simulink model "BuckBoost1"  (Simulink 8.0)
settings: Solver=FixedStepDiscrete  StartTime=0.0  StopTime=5  FixedStep=1e-5  RelTol=1e-3
undefined symbols (not defined in the file): Imax, R, Ts, Vin
libraries: powerlib x12, powerlib_extras x2
settings Model: Creator=zxn  LastModifiedBy=Harri
settings DataIOCC: SignalLoggingSaveFormat=ModelDataLogs
settings DebuggingCC: FcnCallInpInsideContextMsg=UseLocalSettings
settings GRTTargetCC: CombineOutputUpdateFcns=off  GRTInterface=on

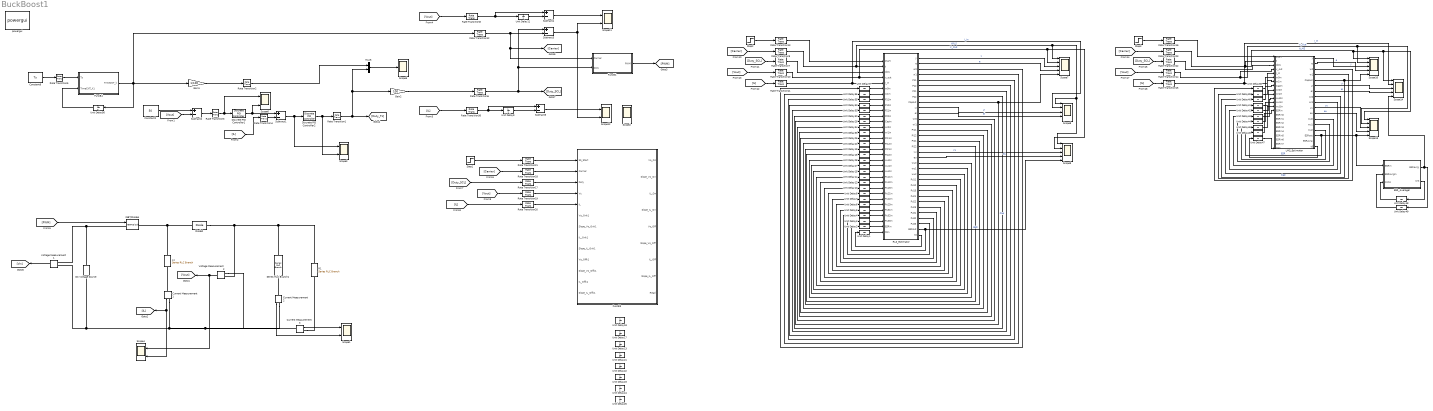
== system BuckBoost1 ==
  Constant2 : Constant  Value=50
  Constant6 : Constant  Value=Ts
  Current Measurement1 : powerlib/Measurements/Current Measurement  PhasorSimulation=off  OutputType=Complex  PSBequivalent=0
  Current Measurement2 : powerlib/Measurements/Current Measurement  PhasorSimulation=off  OutputType=Complex  PSBequivalent=0
  Current Measurement3 : powerlib/Measurements/Current Measurement  PhasorSimulation=off  OutputType=Complex  PSBequivalent=0
  DC Voltage Source : powerlib/Electrical Sources/DC Voltage Source  Amplitude=Vin  Measurements=None
  Diode2 : powerlib/Power Electronics/Diode  Ron=0.001  Lon=0  Vf=0.8  IC=0  UseSnubber=off  Rs=inf  Cs=inf  Measurements=off
  Discrete PID Controller1 : powerlib_extras/Discrete  Control Blocks/Discrete PID Controller  Kp=1.4  Ki=0.4  Kd=0  TcD=0  Par_Limits=[1 -1]*Imax  Init=0  Ts=Ts
  Discrete PID Controller2 : powerlib_extras/Discrete  Control Blocks/Discrete PID Controller  Kp=30e-3  Ki=50e-3  Kd=0  TcD=0  Par_Limits=[1 -1]*0.9  Init=0  Ts=Ts
  ESR_Averager : MATLAB Function  TreatAsAtomicUnit=on
  FuncB1 : MATLAB Function  TreatAsAtomicUnit=on
  FuncB3 : MATLAB Function  TreatAsAtomicUnit=on
  FuncB4 : MATLAB Function  TreatAsAtomicUnit=on
  Gain1 : Gain  Gain=1/100
  Gain2 : Gain  Gain=100
  IGBT/Diode4 : powerlib/Power Electronics/IGBT//Diode  Ron=1e-3  Rs=1e5  Cs=inf  Measurements=off
  L1 : powerlib/Elements/Series RLC Branch  LConnTagsString=__new0  RConnTagsString=__new0  BranchType=L  Resistance=1  Inductance=5e-3  SetiL0=off  InitialCurrent=0  Capacitance=1e-6  Setx0=off  InitialVoltage=0  Measurements=None
  LMS_Estimator : MATLAB Function  TreatAsAtomicUnit=on
  Mux5 : Mux  Inputs=2
  R1 : powerlib/Elements/Series RLC Branch  LConnTagsString=__new0  RConnTagsString=__new0  BranchType=R  Resistance=R  Inductance=1e-3  SetiL0=off  InitialCurrent=0  Capacitance=1e-6  Setx0=off  InitialVoltage=0  Measurements=None
  RLS_Estimator : MATLAB Function  TreatAsAtomicUnit=on
  Rate Transition{1..2,6..23,30} (21 alike) : RateTransition  OutPortSampleTime=1e-5
  Rate Transition3 : RateTransition  OutPortSampleTime=Ts
  Rate Transition4 : RateTransition  OutPortSampleTime=Ts
  Rate Transition5 : RateTransition  X0=Ts  OutPortSampleTime=1e-5
  Scope{1,3..4,6,11..12} (6 alike) : Scope  NumInputPorts=2
      Scope1 settings: TickLabels=on  TimeRange=10  YMin=210~0  YMax=320~47.5  SaveName=var1
      Scope11 settings: TickLabels=on  TimeRange=5  YMin=-0.06~-40  YMax=0.07~65  SaveName=var10  MaxDataPoints=1000000
      Scope12 settings: TickLabels=on  TimeRange=5  YMin=-0.011~-40  YMax=0.01~65  SaveName=var13  MaxDataPoints=1000000
      Scope3 settings: TickLabels=on  TimeRange=1.5  YMin=0.5~0  YMax=0.605~1  SaveName=var4
      Scope4 settings: TickLabels=on  YMin=41.5~2.4  YMax=50~4.3  SaveName=var
      Scope6 settings: TickLabels=on  TimeRange=1.5  YMin=0.5~0  YMax=0.605~1  SaveName=var2
  Scope{7..10,13..14} (6 alike) : Scope  NumInputPorts=5
      Scope10 settings: TickLabels=on  TimeRange=5  YMin=-0.011~-40~-5~-5~-5  YMax=0.01~65~5~5~5  SaveName=var9  MaxDataPoints=1000000
      Scope13 settings: TickLabels=on  TimeRange=5  YMin=-0.011~-40~-5~-5~-5  YMax=0.01~65~5~5~5  SaveName=var11  MaxDataPoints=1000000
      Scope14 settings: TickLabels=on  TimeRange=5  YMin=-0.011~-40~-5~-5~0  YMax=0.01~65~5~5~125  SaveName=var12  MaxDataPoints=1000000
      Scope7 settings: TickLabels=on  TimeRange=5  YMin=-0.011~-40~-5~-5~-5  YMax=0.01~65~5~5~5  SaveName=var6  MaxDataPoints=1000000
      Scope8 settings: TickLabels=on  TimeRange=5  YMin=-0.011~-40~-5~-5~-5  YMax=0.01~65~5~5~5  SaveName=var7  MaxDataPoints=1000000
      Scope9 settings: TickLabels=on  TimeRange=5  YMin=-0.011~-40~-5~-5~-5  YMax=0.01~65~5~5~5  SaveName=var8  MaxDataPoints=1000000
  Scope2 : Scope  NumInputPorts=4
      settings: TickLabels=on  TimeRange=5  YMin=-0.011~-40~-5~-5  YMax=0.01~65~5~5  SaveName=var3  MaxDataPoints=1000000
  Scope5 : Scope
      settings: TickLabels=on  TimeRange=1.5  YMin=0.5  YMax=0.605  SaveName=var5  MaxDataPoints=100000
  Series RLC Branch1 : powerlib/Elements/Series RLC Branch  LConnTagsString=__new0  RConnTagsString=__new0  BranchType=RC  Resistance=80e-3*1  Inductance=1e-3  SetiL0=off  InitialCurrent=0  Capacitance=1e-3*1.75  Setx0=off  InitialVoltage=500  Measurements=None
  Step1 : Step  Time=3.3  SampleTime=0
  Step2 : Step  Time=3.3  SampleTime=0
  Step3 : Step  Time=3.3  SampleTime=0
  Subtract1 : Sum  Inputs=+-  SampleTime=Ts
  Subtract{2..5} (4 alike) : Sum  Inputs=+-
  Unit Delay{1..2,4..6,8..13,15,17..25,27..29,31..34,36..49,56} (43 alike) : UnitDelay  SampleTime=1e-5
  Unit Delay{3,7,14,16,26,30,35} (7 alike) : UnitDelay  InitialCondition=100  SampleTime=1e-5
  Voltage Measurement1 : powerlib/Measurements/Voltage Measurement  PhasorSimulation=off  OutputType=Complex  PSBequivalent=0
  Voltage Measurement2 : powerlib/Measurements/Voltage Measurement  PhasorSimulation=off  OutputType=Complex  PSBequivalent=0
  powergui : powerlib/powergui  Priority=2  SimulationMode=Discrete  SolverType=Tustin  SampleTime=1e-5  frequency=60  SPID=off  DisableSnubberDevices=off  DisableRonSwitches=off  DisableVfSwitches=off  SwTol=0  Interpol=off  DisplayEquations=off  FunctionMessages=off  frequencyindice=0  Pbase=100e6  ErrMax=1e-4  Iterations=50  UnitsV=kV  UnitsW=MW  echomessages=off  HookPort=off  EnableUseOfTLC=off  x0status=blocks  RestoreLinks=warning  ResistiveCurrentMeasurement=off  Frange=[0:2:500]  Ylog=off  Xlog=off  ShowGrid=off  save=off  variable=ZData  structure=ScopeData  ZoomFFT=on  StartTime=0.0  cycles=1  DisplayStyle=1  fundamental=60  FreqAxis=off  MaxFrequency=8000  frequencyindicesteady=1  RmsSteady=1  display=off  Ts=0  methode=off
  wires:
  Constant2/1 -> Subtract2/1
  Subtract2/1 -> Rate Transition3/1
  Voltage Measurement2/1 -> Scope4/1, [Vout]
  Current Measurement1/1 -> [IL], Scope4/2
  Current Measurement3/1 -> Scope1/1
  Current Measurement2/1 -> Scope1/2
  Rate Transition2/1 -> Mux5/1
  Rate Transition3/1 -> Discrete PID Controller1/1, Scope6/1
  Discrete PID Controller1/1 -> Subtract1/1, Scope6/2
  Subtract1/1 -> Discrete PID Controller2/1, Scope3/1
  Rate Transition4/1 -> Subtract1/2
  [IL] -> Rate Transition4/1
  [Vout] -> Subtract2/2
  Discrete PID Controller2/1 -> Rate Transition1/1, Scope3/2
  Rate Transition1/1 -> Mux5/2, Gain2/1, [Duty_Ts]
  Mux5/1 -> Scope5/1
  Rate Transition6/1 -> [Duty_SCL], Subtract3/1, FuncB1/2(Duty)
  Rate Transition8/1 -> Unit Delay11/1, Subtract4/1
  [PWM] -> IGBT/Diode4/1
  Voltage Measurement1/1 -> [Vin]
  Rate Transition5/1 -> FuncB4/1(Ts)
  Constant6/1 -> Rate Transition5/1
  Unit Delay56/1 -> FuncB4/2(TimeCNT_k1)
  FuncB4/1(TimeCNT_k) -> Unit Delay56/1, Gain1/1, Rate Transition12/1
  Gain1/1 -> Rate Transition2/1
  Gain2/1 -> Rate Transition6/1
  Subtract3/1 -> Scope11/2, Scope12/2
  Rate Transition12/1 -> Subtract3/2, [Carrier], FuncB1/1(Carrier)
  Unit Delay11/1 -> Subtract4/2
  Subtract4/1 -> Scope11/1
  [Vout] -> Rate Transition8/1
  [Carrier] -> Rate Transition18/1
  [Duty_SCL] -> Rate Transition17/1
  Step1/1 -> Rate Transition21/1
  [IL] -> Rate Transition20/1
  [Vout] -> Rate Transition19/1
  FuncB1/1(PWM) -> [PWM]
  Rate Transition21/1 -> FuncB3/1(SS_Start)
  Rate Transition18/1 -> FuncB3/2(Carrier)
  Rate Transition17/1 -> FuncB3/3(Duty)
  Rate Transition19/1 -> FuncB3/4(Vc)
  Rate Transition20/1 -> FuncB3/5(IL)
  [IL] -> Rate Transition30/1
  Unit Delay9/1 -> Subtract5/2
  Rate Transition30/1 -> Unit Delay9/1, Subtract5/1
  Subtract5/1 -> Scope12/1
  [Carrier] -> Rate Transition9/1
  [Duty_SCL] -> Rate Transition7/1
  Step2/1 -> Rate Transition13/1
  [IL] -> Rate Transition11/1
  [Vout] -> Rate Transition10/1
  Rate Transition9/1 -> Scope7/1, Scope8/1, Scope9/1, RLS_Estimator/2(t)  "tRLS"
  Rate Transition7/1 -> RLS_Estimator/3(duty)
  Rate Transition10/1 -> Scope7/2, Scope9/2, RLS_Estimator/4(v_out)  "V_Out"
  Rate Transition11/1 -> Scope8/2, RLS_Estimator/5(i_in)  "I_In"
  Rate Transition13/1 -> RLS_Estimator/1(start)
  Unit Delay1/1 -> RLS_Estimator/32(t0in)
  Unit Delay2/1 -> RLS_Estimator/31(ESRin)
  Unit Delay3/1 -> RLS_Estimator/30(Pu33in)
  Unit Delay4/1 -> RLS_Estimator/29(Pu32in)
  Unit Delay5/1 -> RLS_Estimator/28(Pu31in)
  Unit Delay6/1 -> RLS_Estimator/27(Pu23in)
  Unit Delay7/1 -> RLS_Estimator/26(Pu22in)
  Unit Delay8/1 -> RLS_Estimator/25(Pu21in)
  Unit Delay10/1 -> RLS_Estimator/24(Pu13in)
  Unit Delay12/1 -> RLS_Estimator/23(Pu12in)
  Unit Delay14/1 -> RLS_Estimator/22(Pu11in)
  Unit Delay15/1 -> RLS_Estimator/21(wu2in)
  Unit Delay27/1 -> RLS_Estimator/20(wu1in)
  Unit Delay28/1 -> RLS_Estimator/19(wu0in)
  Unit Delay16/1 -> RLS_Estimator/18(Pi22in)
  Unit Delay19/1 -> RLS_Estimator/17(Pi21in)
  Unit Delay20/1 -> RLS_Estimator/16(Pi12in)
  Unit Delay26/1 -> RLS_Estimator/15(Pi11in)
  Unit Delay33/1 -> RLS_Estimator/14(wi1in)
  Unit Delay34/1 -> RLS_Estimator/13(wi0in)
  Unit Delay29/1 -> RLS_Estimator/12(Capin)
  Unit Delay30/1 -> RLS_Estimator/11(P22in)
  Unit Delay31/1 -> RLS_Estimator/10(P21in)
  Unit Delay32/1 -> RLS_Estimator/9(P12in)
  Unit Delay35/1 -> RLS_Estimator/8(P11in)
  Unit Delay36/1 -> RLS_Estimator/7(w1in)
  Unit Delay37/1 -> RLS_Estimator/6(w0in)
  RLS_Estimator/33(t0) -> Unit Delay1/1
  RLS_Estimator/32(ESRout) -> Unit Delay2/1, Scope9/5  "ESR"
  RLS_Estimator/31(Pu33) -> Unit Delay3/1
  RLS_Estimator/30(Pu32) -> Unit Delay4/1
  RLS_Estimator/29(Pu31) -> Unit Delay5/1
  RLS_Estimator/28(Pu23) -> Unit Delay6/1
  RLS_Estimator/27(Pu22) -> Unit Delay7/1
  RLS_Estimator/26(Pu21) -> Unit Delay8/1
  RLS_Estimator/25(Pu13) -> Unit Delay10/1
  RLS_Estimator/24(Pu12) -> Unit Delay12/1
  RLS_Estimator/23(Pu11) -> Unit Delay14/1
  RLS_Estimator/22(wu2) -> Unit Delay15/1
  RLS_Estimator/21(wu1) -> Unit Delay27/1
  RLS_Estimator/20(wu0) -> Unit Delay28/1
  RLS_Estimator/17(Pi22) -> Unit Delay16/1
  RLS_Estimator/16(Pi21) -> Unit Delay19/1
  RLS_Estimator/15(Pi12) -> Unit Delay20/1
  RLS_Estimator/14(Pi11) -> Unit Delay26/1
  RLS_Estimator/13(wi1) -> Unit Delay33/1
  RLS_Estimator/12(wi0) -> Unit Delay34/1
  RLS_Estimator/9(Capout) -> Unit Delay29/1, Scope7/5  "Cap"
  RLS_Estimator/8(P22) -> Unit Delay30/1
  RLS_Estimator/7(P21) -> Unit Delay31/1
  RLS_Estimator/6(P12) -> Unit Delay32/1
  RLS_Estimator/5(P11) -> Unit Delay35/1
  RLS_Estimator/4(w1) -> Unit Delay36/1
  RLS_Estimator/3(w0) -> Unit Delay37/1
  RLS_Estimator/2(e) -> Scope7/4  "e"
  RLS_Estimator/1(y) -> Scope7/3  "y"
  RLS_Estimator/10(yi) -> Scope8/3  "yi"
  RLS_Estimator/11(ei) -> Scope8/4  "ei"
  RLS_Estimator/18(yu) -> Scope9/3  "yu"
  RLS_Estimator/19(eu) -> Scope9/4  "eu"
  [Carrier] -> Rate Transition23/1
  [Duty_SCL] -> Rate Transition22/1
  Step3/1 -> Rate Transition16/1
  [IL] -> Rate Transition15/1
  [Vout] -> Rate Transition14/1
  Rate Transition23/1 -> Scope14/1, Scope13/1, Scope10/1, LMS_Estimator/2(t)  "tLMS"
  Rate Transition22/1 -> LMS_Estimator/3(duty)
  Rate Transition14/1 -> Scope10/2, Scope13/2, LMS_Estimator/4(v_out)  "V_Out"
  Rate Transition15/1 -> Scope14/2, LMS_Estimator/5(i_in)  "I_In"
  Rate Transition16/1 -> LMS_Estimator/1(start)
  Unit Delay47/1 -> LMS_Estimator/23(t0in)
  Unit Delay46/1 -> LMS_Estimator/14(ESRin)
  Unit Delay45/1 -> LMS_Estimator/13(wu2in)
  Unit Delay44/1 -> LMS_Estimator/12(wu1in)
  Unit Delay43/1 -> LMS_Estimator/11(wu0in)
  Unit Delay42/1 -> LMS_Estimator/10(wi1in)
  Unit Delay41/1 -> LMS_Estimator/9(wi0in)
  Unit Delay40/1 -> LMS_Estimator/8(Capin)
  Unit Delay39/1 -> LMS_Estimator/7(w1in)
  Unit Delay38/1 -> LMS_Estimator/6(w0in)
  LMS_Estimator/17(t0) -> Unit Delay47/1
  LMS_Estimator/15(ESRout) -> Unit Delay46/1, ESR_Averager/1(ESRin), Scope13/5  "ESR"
  LMS_Estimator/14(wu2) -> Unit Delay45/1
  LMS_Estimator/13(wu1) -> Unit Delay44/1
  LMS_Estimator/12(wu0) -> Unit Delay43/1
  LMS_Estimator/9(wi1) -> Unit Delay42/1
  LMS_Estimator/8(wi0) -> Unit Delay41/1
  LMS_Estimator/4(w1) -> Unit Delay39/1
  LMS_Estimator/3(w0) -> Unit Delay38/1
  LMS_Estimator/1(y) -> Scope10/3  "y"
  LMS_Estimator/2(e) -> Scope10/4  "e"
  LMS_Estimator/5(Capout) -> Unit Delay40/1, Scope10/5  "Cap"
  LMS_Estimator/6(yi) -> Scope14/3  "yi"
  LMS_Estimator/7(ei) -> Scope14/4  "ei"
  LMS_Estimator/11(eu) -> Scope13/4  "eu"
  LMS_Estimator/10(yu) -> Scope13/3  "yu"
  ESR_Averager/2(Cnt) -> Unit Delay48/1
  Unit Delay48/1 -> ESR_Averager/3(CntIn)
  ESR_Averager/1(ESRavrg) -> Scope14/5, Unit Delay49/1
  Unit Delay49/1 -> ESR_Averager/2(ESRavrgIn)
  connections:
  DC Voltage Source/RConn1 -- IGBT/Diode4/LConn1 -- Voltage Measurement1/LConn1
  Diode2/RConn1 -- IGBT/Diode4/RConn1 -- L1/RConn1
  Current Measurement3/LConn1 -- Current Measurement2/RConn1 -- Voltage Measurement2/LConn1 -- Current Measurement1/RConn1 -- DC Voltage Source/LConn1 -- Voltage Measurement1/LConn2
  Current Measurement1/LConn1 -- L1/LConn1
  Diode2/LConn1 -- R1/RConn1 -- Series RLC Branch1/RConn1 -- Voltage Measurement2/LConn2
  Current Measurement2/LConn1 -- Series RLC Branch1/LConn1
  Current Measurement3/RConn1 -- R1/LConn1

== matlab function RLS_Estimator ==
  data: start input double; t input double; duty input double; v_out input double; i_in input double; w0in input double; w1in input double; P11in input double; P12in input double; P21in input double; P22in input double; Capin input double; y output double; e output double; w0 output double; w1 output double; P11 output double; P12 output double; P21 output double; P22 output double; Capout output double; wi0in input double; wi1in input double; Pi11in input double; Pi12in input double; Pi21in input double; Pi22in input double; wu0in input double; wu1in input double; wu2in input double; Pu11in input double; Pu12in input double; Pu13in input double; Pu21in input double; Pu22in input double; Pu23in input double; Pu31in input double; Pu32in input double; Pu33in input double; ESRin input double; t0in input double; yi output double; ei output double; wi0 output double; wi1 output double; Pi11 output double; Pi12 output double; Pi21 output double; Pi22 output double; yu output double; eu output double; wu0 output double; wu1 output double; wu2 output double; Pu11 output double; Pu12 output double; Pu13 output double; Pu21 output double; Pu22 output double; Pu23 output double; Pu31 output double; Pu32 output double; Pu33 output double; ESRout output double; t0 output double
function [y, e, w0, w1, P11, P12, P21, P22, Capout, ...
    yi, ei, wi0, wi1, Pi11, Pi12, Pi21, Pi22, ...
    yu, eu, wu0, wu1, wu2, Pu11, Pu12, Pu13, Pu21, Pu22, Pu23, Pu31, Pu32, Pu33, ESRout, ...
    t0]  = ...
    Est_RLS(start,t,duty,v_out,i_in, ...
    w0in, w1in, P11in, P12in, P21in, P22in, Capin, ...
    wi0in, wi1in, Pi11in, Pi12in, Pi21in, Pi22in, ...
    wu0in, wu1in, wu2in, Pu11in, Pu12in, Pu13in, Pu21in, Pu22in, Pu23in, Pu31in, Pu32in, Pu33in, ESRin, ...
    t0in)
%#codegen

% *** Time Partition ******************************************************
sampling_time = 1e-5;% 1e-6;

offset = t - duty;

OFFSET_ON_START_abs = 0+5; % for t
OFFSET_ON_END_rel = -5; % for offset
OFFSET_OFF_START_rel = 5; % for offset
OFFSET_OFF_END_abs = 90+5; % for t
% --- end of Time Partition -----------------------------------------------

% *** Init ****************************************************************
lambda = 0.6;
% good for change: 0.7; not good with change: 0.999;
delta = 1/100;

% <<~~~ uON(t) = w0 + w1*t ~~~~~~~~~~~~~~~~~~~~~~~~~~~~~~~~~~~~~~~~~~~~~~>>

% ... estimator output ...
y = 0.0;
e = 0.0;

% ... inputs ...
u = transpose(zeros(1,2));
u(1) = 1;
u(2) = t;

% ... coefficients ...
w = zeros(2,1);
w(1) = w0in;
w(2) = w1in;
w0 = w0in; w1 = w1in;

% ... algorithm specific tools ...
P = eye(2) / delta;
P(1,1) = P11in; P(1,2) = P12in;
P(2,1) = P21in; P(2,2) = P22in;
%NOTE: in "delay unit" blocks, set:
% P11in and P22in --> 100 (as per 'delta')
% P12in and P21in --> 0 (since "eye" matrix)
P11 = P11in; P12 = P12in;
P21 = P21in; P22 = P22in;

% <<~~~ iLOFF(t) = wi0 + wi1*t ~~~~~~~~~~~~~~~~~~~~~~~~~~~~~~~~~~~~~~~~~~>>

% ... estimator output ...
yi = 0.0;
ei = 0.0;

% ... inputs ...
% REUSE

% ... coefficients ...
wi = zeros(2,1);
wi(1) = wi0in;
wi(2) = wi1in;
wi0 = wi0in; wi1 = wi1in;

% ... algorithm specific tools ...
Pi = eye(2) / delta;
Pi(1,1) = Pi11in; Pi(1,2) = Pi12in;
Pi(2,1) = Pi21in; Pi(2,2) = Pi22in;
%NOTE: in "delay unit" blocks, set:
% P11in and P22in --> 100 (as per 'delta')
% P12in and P21in --> 0 (since "eye" matrix)
Pi11 = Pi11in; Pi12 = Pi12in;
Pi21 = Pi21in; Pi22 = Pi22in;

% <<~~~ uON(t) = wu0 + wu1*t + wu2*t^2 ~~~~~~~~~~~~~~~~~~~~~~~~~~~~~~~~~~>>

% ... estimator output ...
yu = 0.0;
eu = 0.0;

% ... inputs ...
uu = transpose(zeros(1,3));
uu(1) = 1;
uu(2) = t;
uu(3) = t*t;

% ... coefficients ...
wu = zeros(3,1);
wu(1) = wu0in;
wu(2) = wu1in;
wu(3) = wu2in;
wu0 = wu0in; wu1 = wu1in; wu2 = wu2in;

% ... algorithm specific tools ...
Pu = eye(3) / delta;
% TODO: remove P(i,j) with i!=j...
Pu(1,1) = Pu11in; Pu(1,2) = Pu12in; Pu(1,3) = Pu13in;
Pu(2,1) = Pu21in; Pu(2,2) = Pu22in; Pu(2,3) = Pu23in;
Pu(3,1) = Pu31in; Pu(3,2) = Pu32in; Pu(3,3) = Pu33in;
%NOTE: in "delay unit" blocks, set:
% P11in and P22in --> 100 (as per 'delta')
% P12in and P21in --> 0 (since "eye" matrix)
Pu11 = Pu11in; Pu12 = Pu12in; Pu13 = Pu13in;
Pu21 = Pu21in; Pu22 = Pu22in; Pu23 = Pu23in;
Pu31 = Pu31in; Pu32 = Pu32in; Pu33 = Pu33in;

% --- end of Init ---------------------------------------------------------

% *** Misc. ***************************************************************

Capout = Capin;
ESRout = ESRin;
t0 = t0in;

% --- end of Misc. --------------------------------------------------------

noiseAmp = 0; % rand : [0,1]

if(start==1)
    % *** State: ON *******************************************************
    if(t > OFFSET_ON_START_abs && offset < OFFSET_ON_END_rel) % ON
        % estimate the "C"
        if(t > OFFSET_ON_START_abs && t<= OFFSET_ON_START_abs+2)
            t0 = t;
        else
            % --- start of RLS for uON(t) ---
            %u(2) = t - t0; NOTE: RLS do not require this kind of offsetting!
            u(2) = (t - t0) * sampling_time; %NOTE: not necessary to offset!
            k = ( (P*u) / (1 + (u' * P * u) / lambda) ) / lambda;
            y = w' * u;
            %e = v_out - y;
            e = (v_out + (noiseAmp*rand)) - y;

            w = w + k*e;
            w0 = w(1); w1 = w(2);

            P = ( P - k * u' * P ) / lambda;
            P11 = P(1,1); P12 = P(1,2);
            P21 = P(2,1); P22 = P(2,2);
            % --- end of RLS for uON(t) ---
        end
    end
    if(offset >= OFFSET_ON_END_rel && offset <= OFFSET_ON_END_rel+1)
        Capout = -w0/w1/30;%*sampling_time;%R=30
    end
    % --- end State: ON ---------------------------------------------------
    
    % *** State: OFF ******************************************************
    if(offset > OFFSET_OFF_START_rel && t < OFFSET_OFF_END_abs) % OFF
        % estimate the "ESR"
        if(offset > OFFSET_OFF_START_rel && offset <= OFFSET_OFF_START_rel+2)
            t0 = t;
        else
            % --- start RLS for iLOFF(t) ---
            u(2) = (t - t0) * sampling_time; %NOTE: not necessary to offset!
            k = ( (Pi*u) / (1 + (u' * Pi * u) / lambda) ) / lambda;
            yi = wi' * u;
            %ei = i_in - yi;
            ei = (i_in + (noiseAmp*rand)) - yi;

            wi = wi + k*ei;
            wi0 = wi(1); wi1 = wi(2);

            Pi = ( Pi - k * u' * Pi ) / lambda;
            Pi11 = Pi(1,1); Pi12 = Pi(1,2);
            Pi21 = Pi(2,1); Pi22 = Pi(2,2);
            % --- end of RLS for iLOFF(t) ---

            % --- start RLS for uOFF(t) ---
            uu(2) = (t - t0) * sampling_time; %NOTE: not necessary to offset!
            uu(3) = uu(2)*uu(2);
            ku = ( (Pu*uu) / (1 + (uu' * Pu * uu) / lambda) ) / lambda;
            yu = wu' * uu;
            %eu = v_out - yu;
            eu = (v_out + (noiseAmp*rand)) - yu;

            wu = wu + ku*eu;
            wu0 = wu(1); wu1 = wu(2); wu2 = wu(3);

            Pu = ( Pu - ku * uu' * Pu ) / lambda;
            Pu11 = Pu(1,1); Pu12 = Pu(1,2); Pu13 = Pu(1,3);
            Pu21 = Pu(2,1); Pu22 = Pu(2,2); Pu23 = Pu(2,3);
            Pu31 = Pu(3,1); Pu32 = Pu(3,2); Pu33 = Pu(3,3);
            % --- end of RLS for uOFF(t) ---
        end
    end
    if(t >= OFFSET_OFF_END_abs && t <= OFFSET_OFF_END_abs+1)
        a = 2*wu2 / (wi1*30 - wu1);
        b = 2*wu2 / (1 - wu1/30/wi1);
        c = wu0*a + b/a - 2*wu2/a;
        ESRout = (wi0/Capin - c) / (c/30 - wi1);
    end
    % --- end State: OFF --------------------------------------------------

end

== matlab function FuncB3 ==
  data: SS_Start input double; Carrier input double; Duty input double; Vc input double; IL input double; Vo_Onk1 input double; Slope_Vo_Onk1 input double; IL_Onk1 input double; Slope_IL_Onk1 input double; Vo_Offk1 input double; Slope_Vo_Offk1 input double; IL_Offk1 input double; Vo_On output double; Slope_Vo_On output double; IL_On output double; Slope_IL_On output double; Vo_Off output double; Slope_Vo_Off output double; IL_Off output double; Slope_IL_Off output double; Read output double; Slope_IL_Offk1 input double
function [Vo_On,Slope_Vo_On,IL_On,Slope_IL_On,Vo_Off,Slope_Vo_Off,IL_Off,Slope_IL_Off,Read] = Sample(SS_Start,Carrier,Duty,Vc,IL,Vo_Onk1,Slope_Vo_Onk1,IL_Onk1,Slope_IL_Onk1,Vo_Offk1,Slope_Vo_Offk1,IL_Offk1,Slope_IL_Offk1)

Err1=(Carrier - Duty);  Tsimulation=1e-5;%1e-6;
%DtT_On=Duty*Tsimulation;    DtT_Off=(100 - Duty)*Tsimulation;%%!! 100 should be repaced Correspondingly by CNT_Max
Fix10us=10e-6;
if(SS_Start==1)
    if(Err1>=-12)&&(Err1<-11) %%Just After Switch-On; (Err1>=-2)&&(Err1<-1); (Carrier==3)
        Vo_On=Vc; IL_On=IL;
        Read=0;
        Slope_Vo_On=Slope_Vo_Onk1; Slope_IL_On=Slope_IL_Onk1;
        Slope_Vo_Off=Slope_Vo_Offk1; Slope_IL_Off=Slope_IL_Offk1;
        Vo_Off=Vo_Offk1; IL_Off=IL_Offk1;
    elseif((Err1>=-2)&&(Err1<-1)) %%Next moment Switch-Off
        %Slope_Vo_On=(Vc - Vo_Onk1)/DtT_On; Slope_IL_On=(IL - IL_Onk1)/DtT_On;
        Slope_Vo_On=(Vc - Vo_Onk1)/Fix10us; Slope_IL_On=(IL - IL_Onk1)/Fix10us;
        Vo_On=Vo_Onk1; IL_On=IL_Onk1;
        Slope_Vo_Off=Slope_Vo_Offk1; Slope_IL_Off=Slope_IL_Offk1; Read=0; 
        Vo_Off=Vo_Offk1; IL_Off=IL_Offk1;
    elseif(Carrier==89) %%Just After Switch Off; Carrier==98; (Err1>3)&&(Err1<=4)
        Vo_Off=Vc;  IL_Off=IL;
        Slope_Vo_Off=Slope_Vo_Offk1;  Slope_IL_Off=Slope_IL_Offk1;
        Slope_Vo_On=Slope_Vo_Onk1;  Slope_IL_On=Slope_IL_Onk1; Read=0;
        Vo_On=Vo_Onk1; IL_On=IL_Onk1;
    elseif(Carrier==99) %%Next moment Switch-On
        %Slope_Vo_Off=(Vc - Vo_Offk1)/DtT_Off;  Slope_IL_Off=(IL - IL_Offk1)/DtT_Off;
        Slope_Vo_Off=(Vc - Vo_Offk1)/Fix10us;  Slope_IL_Off=(IL - IL_Offk1)/Fix10us;
        Vo_Off=Vo_Offk1;  IL_Off=IL_Offk1;
        Read=1;
        Slope_Vo_On=Slope_Vo_Onk1; Slope_IL_On=Slope_IL_Onk1;
        Vo_On=Vo_Onk1; IL_On=IL_Onk1;
    else
        Vo_On=Vo_Onk1; Slope_Vo_On=Slope_Vo_Onk1; IL_On=IL_Onk1; Slope_IL_On=Slope_IL_Onk1; %%On_Readk1
        Vo_Off=Vo_Offk1;  Slope_Vo_Off=Slope_Vo_Offk1;  IL_Off=IL_Offk1;  Slope_IL_Off=Slope_IL_Offk1; Read=0; %%Off_Readk1
    end
else
    Vo_On=49;  Slope_Vo_On=0.5;  IL_On=4;  Slope_IL_On=0.2;
    Vo_Off=50;  Slope_Vo_Off=0.5;  IL_Off=3.8;  Slope_IL_Off=0.2; Read=0;
end

end

== matlab function LMS_Estimator ==
  data: start input double; t input double; duty input double; v_out input double; i_in input double; w0in input double; w1in input double; Capin input double; y output double; e output double; w0 output double; w1 output double; Capout output double; wi0in input double; wi1in input double; wu0in input double; wu1in input double; wu2in input double; ESRin input double; ESRin0 input double; ESRin1 input double; ESRin2 input double; ESRin3 input double; ESRin4 input double; ESRin5 input double; ESRin6 input double; ESRin7 input double; t0in input double; yi output double; ei output double; wi0 output double; wi1 output double; yu output double; eu output double; wu0 output double; wu1 output double; wu2 output double; ESRout output double; ESRavrg output double; t0 output double
function [y, e, w0, w1, Capout, ...
    yi, ei, wi0, wi1, ...
    yu, eu, wu0, wu1, wu2, ESRout, ...
    ESRavrg, ...
    t0]  = ...
    Est_LMS(start,t,duty,v_out,i_in, ...
    w0in, w1in, Capin, ...
    wi0in, wi1in, ...
    wu0in, wu1in, wu2in, ESRin, ...
    ESRin0, ESRin1, ESRin2, ESRin3, ESRin4, ESRin5, ESRin6, ESRin7, ...
    t0in)
%#codegen

% *** Time Partition ******************************************************
sampling_time = 1e-5;% 1e-6;

offset = t - duty;

OFFSET_ON_START_abs = 0+5; % for t
OFFSET_ON_END_rel = -5; % for offset
OFFSET_OFF_START_rel = 5; % for offset
OFFSET_OFF_END_abs = 90+5; % for t
% --- end of Time Partition -----------------------------------------------

% *** Init ****************************************************************
beta = 0.5;

% <<~~~ uON(t) = w0 + w1*t ~~~~~~~~~~~~~~~~~~~~~~~~~~~~~~~~~~~~~~~~~~~~~~>>

% ... estimator output ...
y = 0.0;
e = 0.0;

% ... inputs ...
u = transpose(zeros(1,2));
u(1) = 1;
u(2) = t;

% ... coefficients ...
w = transpose(zeros(1,2));
w(1) = w0in;
w(2) = w1in;
w0 = w0in; w1 = w1in;

% ... algorithm specific tools ...
% none

% <<~~~ iLOFF(t) = wi0 + wi1*t ~~~~~~~~~~~~~~~~~~~~~~~~~~~~~~~~~~~~~~~~~~>>

% ... estimator output ...
yi = 0.0;
ei = 0.0;

% ... inputs ...
% REUSE

% ... coefficients ...
wi = zeros(2,1);
wi(1) = wi0in;
wi(2) = wi1in;
wi0 = wi0in; wi1 = wi1in;

% ... algorithm specific tools ...
% none

% <<~~~ uON(t) = wu0 + wu1*t + wu2*t^2 ~~~~~~~~~~~~~~~~~~~~~~~~~~~~~~~~~~>>

% ... estimator output ...
yu = 0.0;
eu = 0.0;

% ... inputs ...
uu = transpose(zeros(1,3));
uu(1) = 1;
uu(2) = t;
uu(3) = t*t;

% ... coefficients ...
wu = zeros(3,1);
wu(1) = wu0in;
wu(2) = wu1in;
wu(3) = wu2in;
wu0 = wu0in; wu1 = wu1in; wu2 = wu2in;

% ... algorithm specific tools ...
% none

% --- end of Init ---------------------------------------------------------

% *** Misc. ***************************************************************

Capout = Capin;
ESRout = ESRin;
t0 = t0in;

ESRavrg = (ESRin0+ESRin1+ESRin2+ESRin3+ESRin4+ESRin5+ESRin6+ESRin7)/8;

% --- end of Misc. --------------------------------------------------------

noiseAmp = 0; % rand : [0,1]

if(start==1)
    % *** State: ON *******************************************************
    if(t > OFFSET_ON_START_abs && offset < OFFSET_ON_END_rel) % ON
        % estimate the "C"
        %if(t > OFFSET_ON_START_abs && t<= OFFSET_ON_START_abs+2)
        if(t <= OFFSET_ON_START_abs+2)
            t0 = t;
        %else
        end
            % --- start of LMS for uON(t) ---
            u(2) = (t - t0) ;%* sampling_time; 
            rms = (u(1)^2 + u(2)^2)/2;
            y = w' * u;
            %e = v_out - y;
            e = (v_out + (noiseAmp*rand)) - y;

            w = w + beta*e*u/rms;
            w0 = w(1); w1 = w(2);

            % --- end of LMS for uON(t) ---
        %end
    end
    if(offset >= OFFSET_ON_END_rel && offset <= OFFSET_ON_END_rel+1)
        Capout = -w0/w1/30 * sampling_time;% *sampling_time;%R=30
    end
    % --- end State: ON ---------------------------------------------------
    
    % *** State: OFF ******************************************************
    if(offset > OFFSET_OFF_START_rel && t < OFFSET_OFF_END_abs) % OFF
        % estimate the "ESR"
        if(offset > OFFSET_OFF_START_rel && offset <= OFFSET_OFF_START_rel+2)
            t0 = t;
        %else
        end
            % --- start LMS for iLOFF(t) ---
            %u(2) = (t - t0) * sampling_time; 
            u(2) = (t - t0); 
            rms = (u(1)^2 + u(2)^2)/2;
            yi = wi' * u;
            %ei = i_in - yi;
            ei = (i_in + (noiseAmp*rand)) - yi;

            wi = wi + beta*ei*u/rms;
            wi0 = wi(1); wi1 = wi(2);

            % --- end of LMS for iLOFF(t) ---

            % --- start LMS for uOFF(t) ---
            %uu(2) = (t - t0) * sampling_time; 
            uu(2) = (t - t0); 
            uu(3) = uu(2)*uu(2);
            rmsu = (uu(1)^2 + uu(2)^2 + uu(3)^2)/2;%3;
            yu = wu' * uu;
            %eu = v_out - yu;
            eu = (v_out + (noiseAmp*rand)) - yu;

            wu = wu + beta*eu*uu/rmsu;
            wu0 = wu(1); wu1 = wu(2); wu2 = wu(3);

            % --- end of LMS for uOFF(t) ---
        %end
    end
    if(t >= OFFSET_OFF_END_abs && t <= OFFSET_OFF_END_abs+1)
        wu2real = wu2 / sampling_time^2;
        wu1real = wu1 / sampling_time;
        wu0real = wu0;
        wi1real = wi1 / sampling_time;
        wi0real = wi0;
        a = 2*wu2real / (wi1real*30 - wu1real);
        b = 2*wu2real / (1 - wu1real/30/wi1real);
        c = wu0real*a + b/a - 2*wu2real/a;
        ESRout = (wi0real/Capin - c) / (c/30 - wi1real);
    end
    % --- end State: OFF --------------------------------------------------

end

== matlab function ESR_Averager ==
  data: ESRin input double; ESRavrg output double; ESRavrgIn input double; CntIn input double; Cnt output double
function [ESRavrg, Cnt] = ESR_averager(ESRin, ESRavrgIn, CntIn)
%#codegen

Cnt = CntIn + 1;
%Cnt = CntIn;
% if(Cnt >= 100)
%     Cnt = 0;
%     %ESRavrg = 0;
%     ESRavrg = ESRin/100 + ESRavrgIn;
% else
% 
%     %ESRavrg = ESRin/100 + ESRavrgIn;
%     ESRavrg = ESRavrgIn;
% end
if (Cnt < 64*100)
ESRavrg = ( (Cnt-1)/Cnt * ESRavrgIn + ESRin/Cnt );
%Cnt = CntIn + 1;
else
   %ESRavrg = 0;
   %ESRavrg = ESRavrgIn;
   ESRavrg = ( (Cnt-1)/Cnt * ESRavrgIn + ESRin/Cnt );
   %Cnt = 0;
   Cnt = CntIn - 1; % prevent from growing anymore
end

== matlab function FuncB1 ==
  data: PWM output double; Carrier input double; Duty input double
function PWM  = Sample(Carrier,Duty)

Err1=(Duty - Carrier);
%%Single Switch PWM Signal Generation!
if(Err1>0)
    PWM=1;
else
    PWM=0;
end

end

== matlab function FuncB4 ==
  data: Ts input double; TimeCNT_k1 input double; TimeCNT_k output double
function TimeCNT_k  = IabSlope(Ts,TimeCNT_k1)

Tsimulation=1e-5;%1e-6;
CNT_Ts=Ts/Tsimulation - 1; %%100
%%Vap,Vbt Calculation
if(TimeCNT_k1>=CNT_Ts)
    TimeCNT_k=0;
else
    TimeCNT_k=TimeCNT_k1 + 1;
end

end
